simulink model "Simulations_chapter5_method3"  (R2023a)
settings: Solver=ode23s  StartTime=0.0  StopTime=20  RelTol=1e-3  EnableMultiTasking=on
values from neighbouring files (symbols this model uses):
  A = [0 1 0 -1 0; -k/ms -c0/ms 0 c0/ms -1/ms ; 0 0 0 1 0 ; k/mus c0/mus -kt/mus -c0/mus 1/mus ; 0 0 0 0 -1/tau]    [Chapter5_method3.m]
  C = [-k/ms -c0/ms 0 c0/ms -1/ms ; k/mus c0/mus -kt/mus -c0/mus 1/mus]    [Chapter5_method3.m]
  c0 = 68.83    [Chapter5_method3.m]
  c1 = 21    [Chapter5_method3.m]
  Cobs_g = Cz    [Chapter5_method3.m]
  Cobs_p = Cz    [Chapter5_method3.m]
  Dobs_g = zeros(nz,nphi+ny)    [Chapter5_method3.m]
  Dobs_p = zeros(nz,nphi+ny)    [Chapter5_method3.m]
  fc = 28.07    [Chapter5_method3.m]
  Fer0 = 1    [Init_simulations_chapter5_method3.m]
  k0 = 170.4    [Chapter5_method3.m]
  k1 = 218.16    [Chapter5_method3.m]
  ks = 1396    [Chapter5_method3.m]
  kt = 12270    [Chapter5_method3.m]
  L0_g = L(1:nx,1:ny)    [Chapter5_method3.m]
  L1_g = L(nx+1:2*nx,1:ny)    [Chapter5_method3.m]
  L1_p = Lp{1}    [Chapter5_method3.m]
  L2_p = Lp{2}    [Chapter5_method3.m]
  ms = 2.27    [Chapter5_method3.m]
  mus = 0.25    [Chapter5_method3.m]
  rhomax = 1    [Chapter5_method3.m]
  rhomin = 0    [Chapter5_method3.m]
  scenario = input('Which scenario would you like to run: 1, 2 or 3? Answer = ')    [Init_simulations_chapter5_method3.m]
  tau = 43e-3    (= 0.043)    [Chapter5_method3.m]
  Ts = 0.005    [Init_simulations_chapter5_method3.m]
  umax = 0.35    [Init_simulations_chapter5_method3.m]
  umin = 0.1    [Init_simulations_chapter5_method3.m]
  zs0 = 0.001    [Init_simulations_chapter5_method3.m]
  zsdt0 = 0.001    [Init_simulations_chapter5_method3.m]
  zus0 = 0.001    [Init_simulations_chapter5_method3.m]
  zusdt0 = 0.001    [Init_simulations_chapter5_method3.m]
undefined symbols (not defined in the file or in its folder): B2
libraries: simulink x2, cstblocks x2
settings Model: Creator=aestr  LastModifiedBy=senameo
settings SolverCC: AlgebraicLoopSolver=TrustRegion
settings DataIOCC: LimitDataPoints=on  SaveFormat=Array  ReturnWorkspaceOutputs=off
settings OptimizationCC: LifeSpan=inf
settings DebuggingCC: UnconnectedInputMsg=warning  UnconnectedOutputMsg=warning  UnconnectedLineMsg=warning  SFUnexpectedBacktrackingDiag=warning  SFNoUnconditionalDefaultTransitionDiag=warning  SFExecutionAtInitializationDiag=none  ArithmeticOperatorsInVariantConditions=warning
settings HardwareCC: ProdBitPerPointer=32  ProdBitPerSizeT=32  ProdBitPerPtrDiffT=32  ProdLargestAtomicFloat=None  ProdIntDivRoundTo=Undefined  ProdEndianess=Unspecified  ProdWordSize=32  ProdHWDeviceType=32-bit Generic
settings ModelReferenceCC: EnableRefExpFcnMdlSchedulingChecks=on  PropagateSignalLabelsOutOfModel=off
settings SFSimCC: SimUseLocalCustomCode=off  CustomCodeUndefinedFunction=UseInterfaceOnly
settings RTWCC: RTWUseLocalCustomCode=off  DLArmComputeVersion=19.05
settings CodeAppCC: StateflowObjectComments=on
settings GRTTargetCC: TargetLangStandard=C89/C90 (ANSI)
settings ConfigComp: CovMetricSettings=dw  CovSaveCumulativeToWorkspaceVar=on  CovSaveSingleToWorkspaceVar=on  CovExternalEMLEnable=off

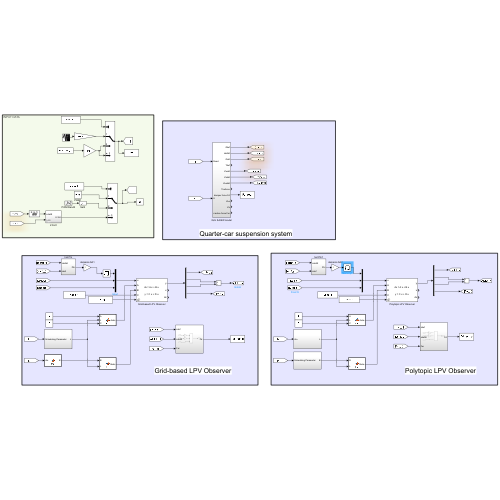
[thumbnail: Simulink's stored preview of the top-level diagram]
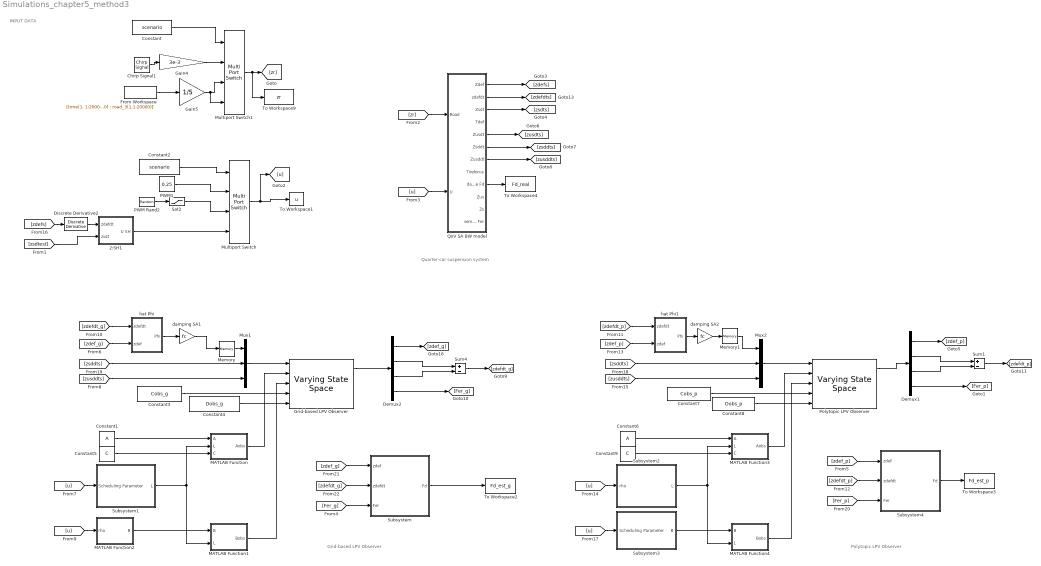
== system Simulations_chapter5_method3 ==
  note: INPUT DATA
  note: Quarter-car suspension system
  note: Grid-based LPV Observer
  note: Polytopic LPV Observer
  2:SH1 : Subsystem  AncestorBlock=controladores/Hybrid Controller/Sky Hook
  Chirp Signal1 : simulink/Sources/Chirp Signal  f1=0  T=20  f2=10
  Constant : Constant  Value=scenario
  Constant1 : Constant  Value=A
  Constant2 : Constant  Value=scenario
  Constant3 : Constant  Value=Cobs_g
  Constant4 : Constant  Value=Dobs_g
  Constant5 : Constant  Value=C
  Constant6 : Constant  Value=A  SampleTime=Ts
  Constant7 : Constant  Value=Cobs_p  SampleTime=Ts
  Constant8 : Constant  Value=Dobs_p  SampleTime=Ts
  Constant9 : Constant  Value=C  SampleTime=Ts
  Demux1 : Demux
  Demux2 : Demux
  Discrete Derivative2 : simulink/Discrete/Discrete Derivative  gainval=1.0  ICPrevScaledInput=0.0  OutMin=[]  OutMax=[]  OutDataType=fixdt(1, 16)  OutScaling=2^-10  DoSatur=off
  From Workspace : FromWorkspace  VariableName=[time(1, 1:20000) ; road_3(1,1:20000)]'
  Gain4 : Gain  Gain=3e-3
  Gain5 : Gain  Gain=1/5
  Grid-based LPV Observer : cstblocks/Linear Parameter Varying/Varying State Space  x0=xobs_0  xNames=''  OutputX=on  OutputDX=on  Feedthrough=on
  MATLAB Function : MATLAB Function  TreatAsAtomicUnit=on
  MATLAB Function1 : MATLAB Function  TreatAsAtomicUnit=on
  MATLAB Function2 : MATLAB Function  TreatAsAtomicUnit=on
  MATLAB Function3 : MATLAB Function  TreatAsAtomicUnit=on
  MATLAB Function4 : MATLAB Function  TreatAsAtomicUnit=on
  Memory : Memory
  Memory1 : Memory
  Multiport Switch : MultiPortSwitch  SaturateOnIntegerOverflow=off  InputSameDT=off
  Multiport Switch1 : MultiPortSwitch  SaturateOnIntegerOverflow=off  InputSameDT=off
  Mux1 : Mux  Inputs=3
  Mux2 : Mux  Inputs=3
  PWM Rand2 : UniformRandomNumber  Minimum=0.05  Maximum=0.4  Seed=5  SampleTime=2
  PWM1 : Constant  Value=0.25
  Polytopic LPV Observer : cstblocks/Linear Parameter Varying/Varying State Space  x0=xobs_0  xNames=''  OutputX=on  OutputDX=on  Feedthrough=on
  QoV SA BW model : Subsystem
  Sat2 : Saturate  UpperLimit=0.35  LowerLimit=0.1
  Subsystem : Subsystem
  Subsystem1 : Subsystem
  Subsystem2 : Subsystem
  Subsystem3 : Subsystem
  Subsystem4 : Subsystem
  Sum1 : Sum  Inputs=+-
  Sum4 : Sum  Inputs=+-
  To Workspace1 : ToWorkspace  VariableName=u  SaveFormat=Structure With Time  SampleTime=Ts
  To Workspace2 : ToWorkspace  VariableName=Fd_est_g  SaveFormat=Structure With Time  SampleTime=-1
  To Workspace3 : ToWorkspace  VariableName=Fd_est_p  SaveFormat=Structure With Time  SampleTime=-1
  To Workspace4 : ToWorkspace  VariableName=Fd_real  SaveFormat=Structure With Time  SampleTime=-1
  To Workspace9 : ToWorkspace  VariableName=zr  SaveFormat=Structure With Time  SampleTime=-1
  damping SA1 : Gain  Gain=fc
  damping SA2 : Gain  Gain=fc
  hat Phi : Subsystem
  hat Phi1 : Subsystem
  wires:
  QoV SA BW model/3(Zsdt) -> [zsdts]
  QoV SA BW model/5(Zusdt) -> [zusdts]
  QoV SA BW model/9(damper force Fd) -> To Workspace4/1
  QoV SA BW model/2(zdefdt) -> [zdefdts]
  QoV SA BW model/1(Zdef) -> [zdefs]
  Multiport Switch1/1 -> To Workspace9/1, [zr]
  Chirp Signal1/1 -> Gain4/1
  [zr] -> QoV SA BW model/1(Road)
  [u] -> QoV SA BW model/2(U)
  [zdefs] -> Discrete Derivative2/1
  Discrete Derivative2/1 -> 2:SH1/1(zdefdt)
  [zsdtest] -> 2:SH1/2(zsdt)
  Constant2/1 -> Multiport Switch/1
  Sat2/1 -> Multiport Switch/3
  PWM1/1 -> Multiport Switch/2
  Multiport Switch/1 -> To Workspace1/1, [u]
  2:SH1/1(U SH) -> Multiport Switch/4
  PWM Rand2/1 -> Sat2/1
  Constant/1 -> Multiport Switch1/1
  Gain4/1 -> Multiport Switch1/2
  From Workspace/1 -> Gain5/1
  Gain5/1 -> Multiport Switch1/4, Multiport Switch1/3
  [u] -> Subsystem2/1(rho)
  [zusddts] -> Mux1/3
  [zdefdt_p] -> hat Phi1/1(zdefdt)
  [zdef_g] -> hat Phi/2(zdef)
  Constant4/1 -> Grid-based LPV Observer/5
  Constant6/1 -> MATLAB Function3/1(A)
  MATLAB Function2/1(B) -> MATLAB Function1/1(B)
  Constant3/1 -> Grid-based LPV Observer/4
  Subsystem/1(Fd) -> To Workspace2/1
  [zdef_p] -> hat Phi1/2(zdef)
  Constant9/1 -> MATLAB Function3/3(C)
  Constant1/1 -> MATLAB Function/1(A)
  hat Phi1/1(Phi) -> damping SA2/1
  [zdefdt_g] -> hat Phi/1(zdefdt)
  Subsystem2/1(L) -> MATLAB Function3/2(L), MATLAB Function4/2(L)
  [zsddts] -> Mux2/2
  Mux2/1 -> Polytopic LPV Observer/1
  [zusddts] -> Mux2/3
  Sum4/1 -> [zdefdt_g]
  MATLAB Function/1(Aobs) -> Grid-based LPV Observer/2
  Subsystem1/1(L) -> MATLAB Function/2(L), MATLAB Function1/2(L)
  Demux2/3 -> Sum4/2
  [u] -> Subsystem3/1(Scheduling Parameter)
  MATLAB Function4/1(Bobs) -> Polytopic LPV Observer/3
  MATLAB Function3/1(Aobs) -> Polytopic LPV Observer/2
  Constant5/1 -> MATLAB Function/3(C)
  Demux2/4 -> [Fer_g]
  Demux2/2 -> Sum4/1
  MATLAB Function1/1(Bobs) -> Grid-based LPV Observer/3
  hat Phi/1(Phi) -> damping SA1/1
  Demux2/1 -> [zdef_g]
  [zsddts] -> Mux1/2
  [u] -> MATLAB Function2/1(rho)
  Constant7/1 -> Polytopic LPV Observer/4
  [u] -> Subsystem1/1(Scheduling Parameter)
  Mux1/1 -> Grid-based LPV Observer/1
  Constant8/1 -> Polytopic LPV Observer/5
  Grid-based LPV Observer/1 -> Demux2/1
  [zdef_g] -> Subsystem/1(zdef)
  [zdefdt_g] -> Subsystem/2(zdefdt)
  [Fer_g] -> Subsystem/3(Fer)
  Polytopic LPV Observer/1 -> Demux1/1
  Demux1/1 -> [zdef_p]
  Demux1/4 -> [Fer_p]
  Subsystem4/1(Fd) -> To Workspace3/1
  Demux1/3 -> Sum1/2
  Demux1/2 -> Sum1/1
  [Fer_p] -> Subsystem4/3(Fer)
  [zdef_p] -> Subsystem4/1(zdef)
  [zdefdt_p] -> Subsystem4/2(zdefdt)
  Sum1/1 -> [zdefdt_p]
  Subsystem3/1(B) -> MATLAB Function4/1(B)
  QoV SA BW model/6(Zsddt) -> [zsddts]
  QoV SA BW model/7(Zusddt) -> [zusddts]
  damping SA1/1 -> Memory/1
  damping SA2/1 -> Memory1/1
  Memory/1 -> Mux1/1
  Memory1/1 -> Mux2/1

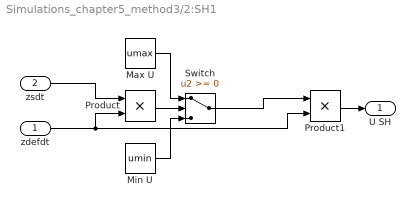
== system Simulations_chapter5_method3/2:SH1 ==
  zdefdt : Inport
  zsdt : Inport  Port=2
  Max U : Constant  Value=umax
  Min U : Constant  Value=umin
  Product : Product  RndMeth=Zero
  Product1 : Product  RndMeth=Zero
  Switch : Switch  SaturateOnIntegerOverflow=off  InputSameDT=off
  U SH : Outport  VectorParamsAs1DForOutWhenUnconnected=off
  wires:
  zsdt/1 -> Product/1
  zdefdt/1 -> Product1/2, Product/2
  Max U/1 -> Switch/1
  Min U/1 -> Switch/3
  Product/1 -> Switch/2
  Switch/1 -> Product1/1
  Product1/1 -> U SH/1

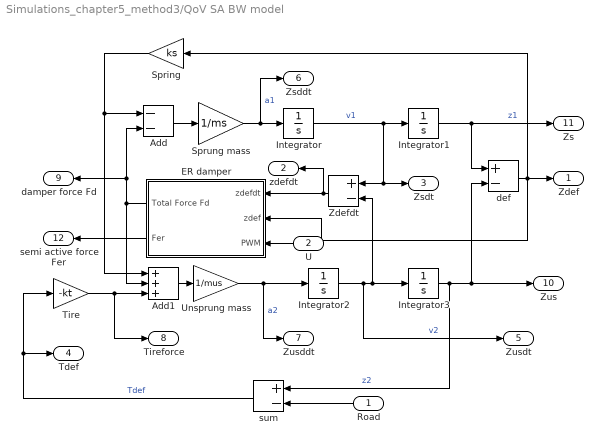
== system Simulations_chapter5_method3/QoV SA BW model ==
  Road : Inport
  U : Inport  Port=2
  Add : Sum  Inputs=--
  Add1 : Sum  Inputs=+++
  ER damper : Subsystem
  Integrator : Integrator  InitialCondition=zsdt0
  Integrator1 : Integrator  InitialCondition=zs0
  Integrator2 : Integrator  InitialCondition=zusdt0
  Integrator3 : Integrator  InitialCondition=zus0
  Spring : Gain  Gain=ks
  Sprung mass : Gain  Gain=1/ms
  Tire : Gain  Gain=-kt
  Unsprung mass : Gain  Gain=1/mus
  Zdefdt : Sum  Inputs=+-
  def : Sum  Inputs=+-
  sum : Sum  Inputs=+-
  Zdef : Outport
  zdefdt : Outport  Port=2
  Zsdt : Outport  Port=3
  Tdef : Outport  Port=4
  Zusdt : Outport  Port=5
  Zsddt : Outport  Port=6
  Zusddt : Outport  Port=7
  Tireforce : Outport  Port=8
  damper force Fd : Outport  Port=9
  Zus : Outport  Port=10
  Zs : Outport  Port=11
  semi active force Fer : Outport  Port=12
  wires:
  Integrator/1 -> Zsdt/1, Zdefdt/1, Integrator1/1  "v1"
  Integrator2/1 -> Zusdt/1, Zdefdt/2, Integrator3/1  "v2"
  Sprung mass/1 -> Zsddt/1, Integrator/1  "a1"
  Unsprung mass/1 -> Zusddt/1, Integrator2/1  "a2"
  Add/1 -> Sprung mass/1
  Add1/1 -> Unsprung mass/1
  Integrator1/1 -> def/1, Zs/1  "z1"
  Integrator3/1 -> sum/1, def/2, Zus/1  "z2"
  def/1 -> ER damper/2(zdef), Zdef/1, Spring/1
  Spring/1 -> Add/1, Add1/1
  Tire/1 -> Tireforce/1, Add1/3
  Road/1 -> sum/2
  sum/1 -> Tdef/1, Tire/1  "Tdef"
  ER damper/1(Total Force Fd) -> Add1/2, Add/2, damper force Fd/1
  U/1 -> ER damper/3(PWM)
  Zdefdt/1 -> ER damper/1(zdefdt), zdefdt/1
  ER damper/2(Fer) -> semi active force Fer/1

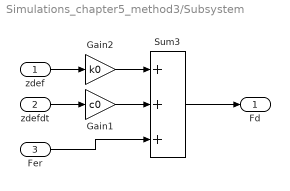
== system Simulations_chapter5_method3/Subsystem ==
  zdef : Inport
  zdefdt : Inport  Port=2
  Fer : Inport  Port=3
  Gain1 : Gain  Gain=c0
  Gain2 : Gain  Gain=k0
  Sum3 : Sum  Inputs=+++
  Fd : Outport
  wires:
  zdef/1 -> Gain2/1
  Gain2/1 -> Sum3/1
  Sum3/1 -> Fd/1
  zdefdt/1 -> Gain1/1
  Gain1/1 -> Sum3/2
  Fer/1 -> Sum3/3

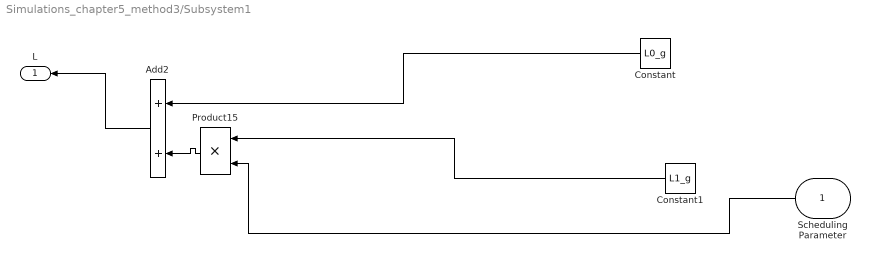
== system Simulations_chapter5_method3/Subsystem1 ==
  Scheduling Parameter : Inport
  Add2 : Sum
  Constant : Constant  Value=L0_g
  Constant1 : Constant  Value=L1_g
  Product15 : Product  RndMeth=Zero
  L : Outport  VectorParamsAs1DForOutWhenUnconnected=off
  wires:
  Scheduling Parameter/1 -> Product15/2
  Add2/1 -> L/1
  Constant/1 -> Add2/1
  Product15/1 -> Add2/2
  Constant1/1 -> Product15/1

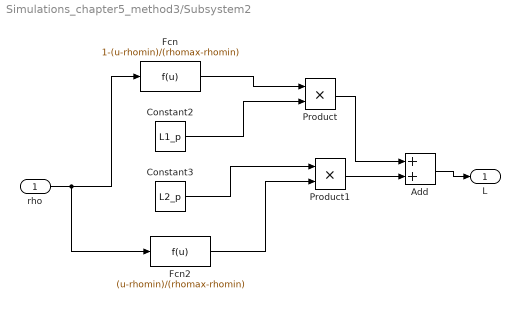
== system Simulations_chapter5_method3/Subsystem2 ==
  rho : Inport
  Add : Sum
  Constant2 : Constant  Value=L1_p  SampleTime=Ts
  Constant3 : Constant  Value=L2_p  SampleTime=Ts
  Fcn : Fcn  Expr=1-(u-rhomin)/(rhomax-rhomin)
  Fcn2 : Fcn  Expr=(u-rhomin)/(rhomax-rhomin)
  Product : Product
  Product1 : Product
  L : Outport  VectorParamsAs1DForOutWhenUnconnected=off
  wires:
  Constant3/1 -> Product1/1
  Fcn/1 -> Product/1
  Fcn2/1 -> Product1/2
  rho/1 -> Fcn/1, Fcn2/1
  Constant2/1 -> Product/2
  Product1/1 -> Add/2
  Product/1 -> Add/1
  Add/1 -> L/1

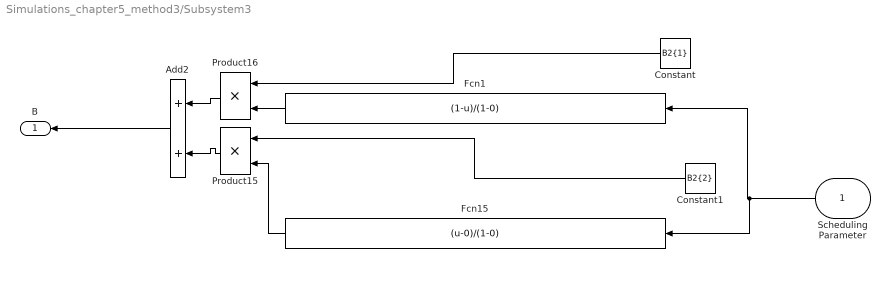
== system Simulations_chapter5_method3/Subsystem3 ==
  Scheduling Parameter : Inport
  Add2 : Sum
  Constant : Constant  Value=B2{1}  SampleTime=Ts
  Constant1 : Constant  Value=B2{2}  SampleTime=Ts
  Fcn1 : Fcn  Expr=(1-u)/(1-0)
  Fcn15 : Fcn  Expr=(u-0)/(1-0)
  Product15 : Product  RndMeth=Zero
  Product16 : Product  RndMeth=Zero
  B : Outport  VectorParamsAs1DForOutWhenUnconnected=off
  wires:
  Fcn1/1 -> Product16/2
  Fcn15/1 -> Product15/2
  Product16/1 -> Add2/1
  Product15/1 -> Add2/2
  Scheduling Parameter/1 -> Fcn15/1, Fcn1/1
  Constant1/1 -> Product15/1
  Constant/1 -> Product16/1
  Add2/1 -> B/1

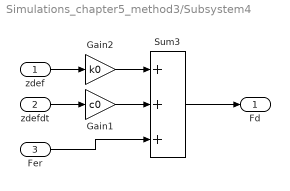
== system Simulations_chapter5_method3/Subsystem4 ==
  zdef : Inport
  zdefdt : Inport  Port=2
  Fer : Inport  Port=3
  Gain1 : Gain  Gain=c0
  Gain2 : Gain  Gain=k0
  Sum3 : Sum  Inputs=+++
  Fd : Outport
  wires:
  zdef/1 -> Gain2/1
  Gain2/1 -> Sum3/1
  Sum3/1 -> Fd/1
  zdefdt/1 -> Gain1/1
  Gain1/1 -> Sum3/2
  Fer/1 -> Sum3/3

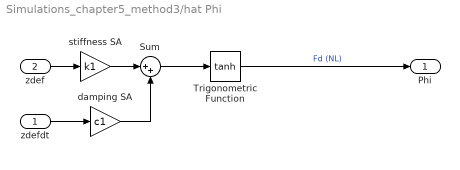
== system Simulations_chapter5_method3/hat Phi ==
  zdefdt : Inport
  zdef : Inport  Port=2
  Sum : Sum  Inputs=|++
  Trigonometric Function : Trigonometry  Operator=tanh
  damping SA : Gain  Gain=c1
  stiffness SA : Gain  Gain=k1
  Phi : Outport  VectorParamsAs1DForOutWhenUnconnected=off
  wires:
  zdefdt/1 -> damping SA/1
  stiffness SA/1 -> Sum/1
  damping SA/1 -> Sum/2
  Sum/1 -> Trigonometric Function/1
  zdef/1 -> stiffness SA/1
  Trigonometric Function/1 -> Phi/1  "Fd (NL)"

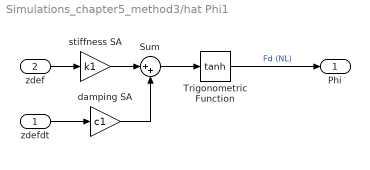
== system Simulations_chapter5_method3/hat Phi1 ==
  zdefdt : Inport
  zdef : Inport  Port=2
  Sum : Sum  Inputs=|++
  Trigonometric Function : Trigonometry  Operator=tanh
  damping SA : Gain  Gain=c1
  stiffness SA : Gain  Gain=k1
  Phi : Outport  VectorParamsAs1DForOutWhenUnconnected=off
  wires:
  zdefdt/1 -> damping SA/1
  stiffness SA/1 -> Sum/1
  damping SA/1 -> Sum/2
  Sum/1 -> Trigonometric Function/1
  zdef/1 -> stiffness SA/1
  Trigonometric Function/1 -> Phi/1  "Fd (NL)"

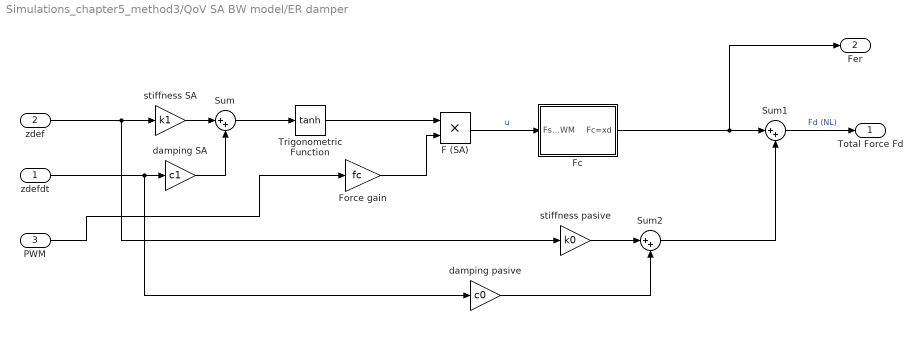
== system Simulations_chapter5_method3/QoV SA BW model/ER damper ==
  zdefdt : Inport
  zdef : Inport  Port=2
  PWM : Inport  Port=3
  "F (SA) " : Product  RndMeth=Zero
  Fc : Subsystem
  Force gain : Gain  Gain=fc
  Sum : Sum  Inputs=|++
  Sum1 : Sum  Inputs=|++
  Sum2 : Sum  Inputs=|++
  Trigonometric Function : Trigonometry  Operator=tanh
  damping SA : Gain  Gain=c1
  damping pasive : Gain  Gain=c0
  stiffness SA : Gain  Gain=k1
  stiffness pasive : Gain  Gain=k0
  Total Force Fd : Outport
  Fer : Outport  Port=2
  wires:
  zdefdt/1 -> damping pasive/1, damping SA/1
  stiffness SA/1 -> Sum/1
  damping SA/1 -> Sum/2
  Sum/1 -> Trigonometric Function/1
  Trigonometric Function/1 -> "F (SA) "/1
  PWM/1 -> Force gain/1
  Force gain/1 -> "F (SA) "/2
  stiffness pasive/1 -> Sum2/1
  damping pasive/1 -> Sum2/2
  "F (SA) "/1 -> Fc/1(Fsa*PWM)  "u"
  Fc/1(Fc=xd) -> Fer/1, Sum1/1
  Sum2/1 -> Sum1/2
  Sum1/1 -> Total Force Fd/1  "Fd (NL)"
  zdef/1 -> stiffness pasive/1, stiffness SA/1

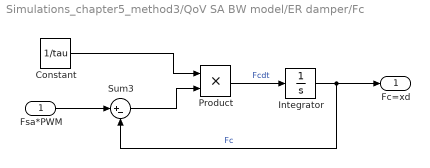
== system Simulations_chapter5_method3/QoV SA BW model/ER damper/Fc ==
  Fsa*PWM : Inport
  Constant : Constant  Value=1/tau
  Integrator : Integrator  InitialCondition=Fer0
  Product : Product  RndMeth=Zero
  Sum3 : Sum  Inputs=|+-
  Fc=xd : Outport
  wires:
  Integrator/1 -> Sum3/2, Fc=xd/1  "Fc"
  Fsa*PWM/1 -> Sum3/1
  Sum3/1 -> Product/2
  Product/1 -> Integrator/1  "Fcdt"
  Constant/1 -> Product/1

== matlab function Simulations_chapter5_method3/MATLAB Function ==
  data: A input; Aobs output; L input; C input
function Aobs = fcn(A,L,C)

 Aobs = A-L*C;

== matlab function Simulations_chapter5_method3/MATLAB Function2 ==
  data: rho input; B output
function B = fcn(rho)
tau=43e-3;
 B = [0 ; 0 ; 0 ; 0 ; rho/tau];

== matlab function Simulations_chapter5_method3/MATLAB Function3 ==
  data: A input; Aobs output; L input; C input
function Aobs = fcn(A,L,C)

 Aobs = A-L*C;

== matlab function Simulations_chapter5_method3/MATLAB Function4 ==
  data: B input; Bobs output; L input
function Bobs = fcn(B,L)

 Bobs = [B,L];

== matlab function Simulations_chapter5_method3/MATLAB Function1 ==
  data: B input; Bobs output; L input
function Bobs = fcn(B,L)

 Bobs = [B,L];
